simulink model "Test1"  (R2021b)
settings: Solver=FixedStepDiscrete  StartTime=0.0  StopTime=inf  RelTol=1e-3
undefined symbols (not defined in the file or in its folder): fdesignblkfcn, gcbh, High
libraries: dspswit3 x3, simulink x2, dspsnks4 x1, dspmtrx3 x1, dspvision x1, dspbuff3 x1, audiosources x1
settings Model: Creator=lenovo  LastModifiedBy=lenovo
settings SolverCC: AlgebraicLoopSolver=TrustRegion  AutoInsertRateTranBlk=on
settings DataIOCC: LimitDataPoints=on  SaveOutput=off  SignalLogging=off  SaveTime=off
settings OptimizationCC: LifeSpan=inf
settings DebuggingCC: AlgebraicLoopMsg=error  SingleTaskRateTransMsg=error  AllowSymbolicDim=off  SFUnexpectedBacktrackingDiag=warning  SFNoUnconditionalDefaultTransitionDiag=warning  SFExecutionAtInitializationDiag=none  SFMachineParentedDataDiag=warning  ArithmeticOperatorsInVariantConditions=warning
settings SFSimCC: SimUseLocalCustomCode=off  CustomCodeUndefinedFunction=UseInterfaceOnly
settings RTWCC: RTWUseLocalCustomCode=off
settings CodeAppCC: StateflowObjectComments=on
settings GRTTargetCC: TargetLangStandard=C89/C90 (ANSI)
settings ConfigComp: CovMetricSettings=dw  CovSaveCumulativeToWorkspaceVar=on  CovSaveSingleToWorkspaceVar=on  CovExternalEMLEnable=off  CovSFcnEnable=off

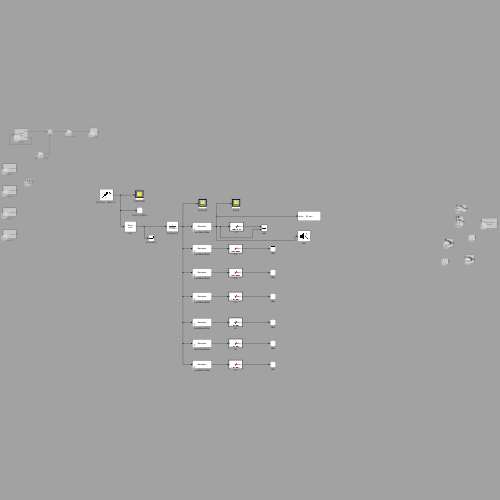
[thumbnail: Simulink's stored preview of the top-level diagram]
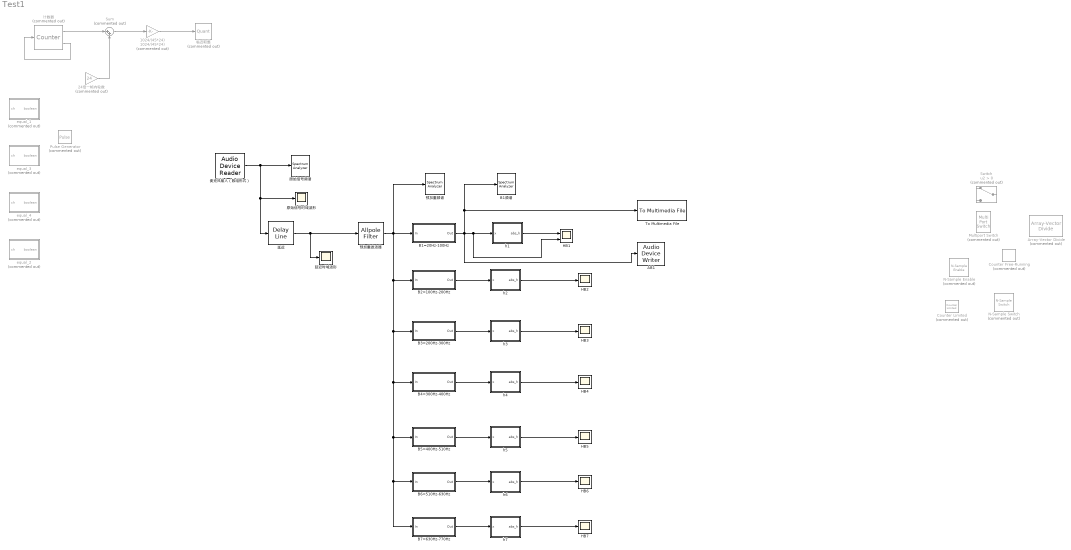
== system Test1 ==
  1024/(45*24) : Gain  Commented=on  Gain=1024/(45*24)
  24倍一帧内轮数 : Gain  Commented=on  Gain=24
  AB1 : dspsnks4/Audio Device Writer  Driver=DirectSound  Device=Default  InheritSampleRate=on  SampleRate=44100  BitDepth=16-bit integer  BufferSize=4096  NumBuffers=10  DefaultOutputChannelMapping=on  OutputChannelMapping=1:2  OutputNumUnderrunSamples=off  DriverIdx=1  DeviceWarnFlag=''
  Array-Vector Divide : dspmtrx3/Array-Vector Divide  Commented=on  Dimension=1  V_Source=Input port  V_VectFromMask=[0.5 0.25]  prodOutputSignedness=Auto  accumSignedness=Auto  roundingMode=Floor  overflowMode=off  firstCoeffSignedness=Auto  firstCoeffDataTypeStr=Inherit: Same word length as input  firstCoeffMin=[]  firstCoeffMax=[]  firstCoeffLastDataTypeStr=Inherit: Same word length as input  outputSignedness=Auto  outputMin=[]  outputMax=[]
      settings: SourceProductBaseCode=DS
  B1=20Hz-100Hz : Subsystem  DialogController=fdesignblkfcn  InitFcn=fdesignblkfcn(gcbh, {'InitFcn'});  mask(Bandpass Filter){}
      mask help: Design a bandpass filter
      settings: CopyFcn=fdesignblkfcn(gcbh, {'CopyFcn'});
      mask Help: helpview(mapfilelocation('dsp'), 'dspbandpassfilter');
      mask Display: disp('Bandpass');
  B1频谱 : SpectrumAnalyzer
  B2=100Hz-200Hz : Subsystem  DialogController=fdesignblkfcn  InitFcn=fdesignblkfcn(gcbh, {'InitFcn'});  mask(Bandpass Filter){}
      mask help: Design a bandpass filter
      settings: CopyFcn=fdesignblkfcn(gcbh, {'CopyFcn'});
      mask Help: helpview(mapfilelocation('dsp'), 'dspbandpassfilter');
      mask Display: disp('Bandpass');
  B3=200Hz-300Hz : Subsystem  DialogController=fdesignblkfcn  InitFcn=fdesignblkfcn(gcbh, {'InitFcn'});  mask(Bandpass Filter){}
      mask help: Design a bandpass filter
      settings: CopyFcn=fdesignblkfcn(gcbh, {'CopyFcn'});
      mask Help: helpview(mapfilelocation('dsp'), 'dspbandpassfilter');
      mask Display: disp('Bandpass');
  B4=300Hz-400Hz : Subsystem  DialogController=fdesignblkfcn  InitFcn=fdesignblkfcn(gcbh, {'InitFcn'});  mask(Bandpass Filter){}
      mask help: Design a bandpass filter
      settings: CopyFcn=fdesignblkfcn(gcbh, {'CopyFcn'});
      mask Help: helpview(mapfilelocation('dsp'), 'dspbandpassfilter');
      mask Display: disp('Bandpass');
  B5=400Hz-510Hz : Subsystem  DialogController=fdesignblkfcn  InitFcn=fdesignblkfcn(gcbh, {'InitFcn'});  mask(Bandpass Filter){}
      mask help: Design a bandpass filter
      settings: CopyFcn=fdesignblkfcn(gcbh, {'CopyFcn'});
      mask Help: helpview(mapfilelocation('dsp'), 'dspbandpassfilter');
      mask Display: disp('Bandpass');
  B6=510Hz-630Hz : Subsystem  DialogController=fdesignblkfcn  InitFcn=fdesignblkfcn(gcbh, {'InitFcn'});  mask(Bandpass Filter){}
      mask help: Design a bandpass filter
      settings: CopyFcn=fdesignblkfcn(gcbh, {'CopyFcn'});
      mask Help: helpview(mapfilelocation('dsp'), 'dspbandpassfilter');
      mask Display: disp('Bandpass');
  B7=630Hz-770Hz : Subsystem  DialogController=fdesignblkfcn  InitFcn=fdesignblkfcn(gcbh, {'InitFcn'});  mask(Bandpass Filter){}
      mask help: Design a bandpass filter
      settings: CopyFcn=fdesignblkfcn(gcbh, {'CopyFcn'});
      mask Help: helpview(mapfilelocation('dsp'), 'dspbandpassfilter');
      mask Display: disp('Bandpass');
  Counter Free-Running : simulink/Sources/Counter Free-Running  Commented=on  NumBits=16  tsamp=-1
  Counter Limited : simulink/Sources/Counter Limited  Commented=on  uplimit=7  tsamp=-1
  HB1 : Scope  NumInputPorts=2
  HB{2..7} (6 alike) : Scope
  Multiport Switch : MultiPortSwitch  Commented=on
  N-Sample Enable : dspswit3/N-Sample Enable  Commented=on  N=8  ActiveLevel=High (1)  reset=off  TriggerType=Rising edge  Ts=1  DataType=Logical
      settings: SourceProductBaseCode=DS
  N-Sample Switch : dspswit3/N-Sample Switch  Commented=on  N=8  reset=off  TriggerType=Rising edge  Ts=0.1
      settings: SourceProductBaseCode=DS
  Pulse Generator : DiscretePulseGenerator  Commented=on  PulseType=Time based  Period=10  PulseWidth=5
  Sum : Sum  Commented=on  Inputs=|++
  Switch : Switch  Commented=on  Criteria=u2 > Threshold
  To Multimedia File : dspvision/To Multimedia File  outputFilename=B1.wav  streamSelection=Audio only  videoCompressor=None (uncompressed)  audioCompressor=None (uncompressed)  imagePorts=Separate color signals  fileType=WAV  audioDatatype=16-bit integer  fourcc=RGB  videoQuality=75  mj2000CompFactor=10
  equal_1 : MATLAB Function  Commented=on  TreatAsAtomicUnit=on
  equal_2 : MATLAB Function  Commented=on  TreatAsAtomicUnit=on
  equal_3 : MATLAB Function  Commented=on  TreatAsAtomicUnit=on
  equal_4 : MATLAB Function  Commented=on  TreatAsAtomicUnit=on
  h1 : MATLAB Function  TreatAsAtomicUnit=on
  h2 : MATLAB Function  TreatAsAtomicUnit=on
  h3 : MATLAB Function  TreatAsAtomicUnit=on
  h4 : MATLAB Function  TreatAsAtomicUnit=on
  h5 : MATLAB Function  TreatAsAtomicUnit=on
  h6 : MATLAB Function  TreatAsAtomicUnit=on
  h7 : MATLAB Function  TreatAsAtomicUnit=on
  临近取整 : Quantizer  Commented=on  QuantizationInterval=1  LinearizeAsGain=off
  原始信号时域波形 : Scope
  原始信号频谱 : SpectrumAnalyzer
  延迟 : dspbuff3/Delay Line  siz=1024  ic=0  directfeed=off  enable_output=off  hold_output=off  OutputFrames=off
      settings: SourceProductBaseCode=DS
  延迟时域波形 : Scope
  计数器 : dspswit3/Counter  Commented=on  Direction=Up  CountEvent=Free running  CounterSize=User defined  MaxCount=25  InitialCount=1  Output=Count and Hit  HitValue=1  ResetInput=on  SamplesPerFrame=24*45  Ts=1/44100  CntDtype=double  HitDtype=Boolean
  预加重滤波器 : AllpoleFilter  Coefficients=[1 -0.95]
  预加重频谱 : SpectrumAnalyzer
  麦克风输入（数组形式） : audiosources/Audio Device Reader  Driver=DirectSound  Device=麦克风阵列 (适用于数字麦克风的英特尔? 智音技术)  SampleRate=44100  NumChannels=1  SamplesPerFrame=1024  BitDepth=16-bit integer  NumBuffers=10  DefaultInputChannelMapping=on  InputChannelMapping=1:2  OutputNumOverrunSamples=off  OutputDataType=double  DriverIdx=1  DeviceWarnFlag=''
      settings: SourceProductBaseCode=AU
  wires:
  麦克风输入（数组形式）/1 -> 原始信号时域波形/1, 延迟/1, 原始信号频谱/1
  延迟/1 -> 延迟时域波形/1, 预加重滤波器/1
  B1=20Hz-100Hz/1(Out) -> AB1/1, HB1/2, h1/1(x), B1频谱/1, To Multimedia File/1
  h1/1(abs_h) -> HB1/1
  B2=100Hz-200Hz/1(Out) -> h2/1(x)
  B3=200Hz-300Hz/1(Out) -> h3/1(x)
  B4=300Hz-400Hz/1(Out) -> h4/1(x)
  B5=400Hz-510Hz/1(Out) -> h5/1(x)
  B6=510Hz-630Hz/1(Out) -> h6/1(x)
  B7=630Hz-770Hz/1(Out) -> h7/1(x)
  h2/1(abs_h) -> HB2/1
  h3/1(abs_h) -> HB3/1
  h4/1(abs_h) -> HB4/1
  h5/1(abs_h) -> HB5/1
  h6/1(abs_h) -> HB6/1
  h7/1(abs_h) -> HB7/1
  计数器/2 -> 计数器/1
  计数器/1 -> Sum/1
  24倍一帧内轮数/1 -> Sum/2
  Sum/1 -> 1024/(45*24)/1
  1024/(45*24)/1 -> 临近取整/1
  预加重滤波器/1 -> B7=630Hz-770Hz/1(In), B6=510Hz-630Hz/1(In), B5=400Hz-510Hz/1(In), B4=300Hz-400Hz/1(In), B3=200Hz-300Hz/1(In), B2=100Hz-200Hz/1(In), 预加重频谱/1, B1=20Hz-100Hz/1(In)

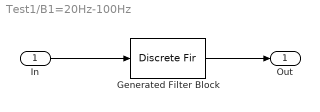
== system Test1/B1=20Hz-100Hz ==
  In : Inport
  Generated Filter Block : DiscreteFir  Tag=BlockMethodSubSystem  Coefficients=[0.00457402244520528894 0.00508602619083937946 0.00659269331412791308 0.00903956144930821194 0.0123353711920271541 0.016355548458740897 0.0209470008592822429 0.0259340418292448825 0.0311252113312927223 0.0363207260934495305 0.0413202670506143815 0.0459307979165471392 0.0499741072000983652 0.0532937765702380661 0.0557613008604806379 0.0572811183038447469 0.0577943524869048084 0.0572811183038447469 0.0557613008604806379 0.0532937765702380661 0.0499741072000983652 0.0459307979165471392 0.0413202670506143815 0.0363207260934495305 0.0311252113312927223 0.0259340418292448825 0.0209470008592822429 0.016355548458740897 0.0123353711920271541 0.00903956144930821194 0.00659269331412791308 0.00508602619083937946 0.00457402244520528894]  InputProcessing=Columns as channels (frame based)
  Out : Outport  VectorParamsAs1DForOutWhenUnconnected=off
  wires:
  In/1 -> Generated Filter Block/1
  Generated Filter Block/1 -> Out/1

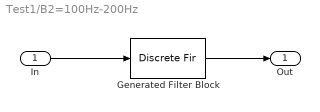
== system Test1/B2=100Hz-200Hz ==
  In : Inport
  Generated Filter Block : DiscreteFir  Tag=BlockMethodSubSystem  Coefficients=[0.00441727693112917499 0.0049428047170021602 0.00644474326614278507 0.00888485385185234372 0.0121851336333958435 0.0162306434727095723 0.0208739501835365493 0.0259410032521986307 0.0312382012424146337 0.0365603488452490091 0.0416991643701427883 0.0464519713170962745 0.0506301977683168147 0.0540673141973552276 0.0566258636594231327 0.0582032771897738541 0.0587362198811968786 0.0582032771897738541 0.0566258636594231327 0.0540673141973552276 0.0506301977683168147 0.0464519713170962745 0.0416991643701427883 0.0365603488452490091 0.0312382012424146337 0.0259410032521986307 0.0208739501835365493 0.0162306434727095723 0.0121851336333958435 0.00888485385185234372 0.00644474326614278507 0.0049428047170021602 0.00441727693112917499]  InputProcessing=Columns as channels (frame based)
  Out : Outport  VectorParamsAs1DForOutWhenUnconnected=off
  wires:
  In/1 -> Generated Filter Block/1
  Generated Filter Block/1 -> Out/1

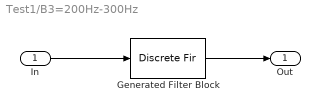
== system Test1/B3=200Hz-300Hz ==
  In : Inport
  Generated Filter Block : DiscreteFir  Tag=BlockMethodSubSystem  Coefficients=[0.0040814662241728597 0.00463418043527237707 0.00612377247553548727 0.00854634110797388227 0.0118523009197635167 0.0159476618531074477 0.02069756837227818 0.0259319465742560012 0.0314529964840676579 0.0370441687734499453 0.0424801854503906937 0.0475376069779057803 0.0520054168949762724 0.0556950910760549422 0.0584496425706742123 0.0601511833336923971 0.060726618501989918 0.0601511833336923971 0.0584496425706742123 0.0556950910760549422 0.0520054168949762724 0.0475376069779057803 0.0424801854503906937 0.0370441687734499453 0.0314529964840676579 0.0259319465742560012 0.02069756837227818 0.0159476618531074477 0.0118523009197635167 0.00854634110797388227 0.00612377247553548727 0.00463418043527237707 0.0040814662241728597]  InputProcessing=Columns as channels (frame based)
  Out : Outport  VectorParamsAs1DForOutWhenUnconnected=off
  wires:
  In/1 -> Generated Filter Block/1
  Generated Filter Block/1 -> Out/1

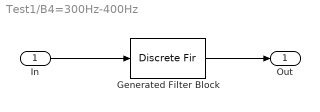
== system Test1/B4=300Hz-400Hz ==
  In : Inport
  Generated Filter Block : DiscreteFir  Tag=BlockMethodSubSystem  Coefficients=[0.00355254435048634127 0.00414283836891639941 0.00560631324623054542 0.0079917846773801017 0.0112942797519545203 0.0154535136154739811 0.0203556333711287542 0.0258381626345098731 0.031697887414365189 0.0377012460605533825 0.0435966336799673629 0.0491279139259522268 0.0540483555780169253 0.0581341824796804546 0.0611969450154634734 0.0630939882821951181 0.0637364024848837418 0.0630939882821951181 0.0611969450154634734 0.0581341824796804546 0.0540483555780169253 0.0491279139259522268 0.0435966336799673629 0.0377012460605533825 0.031697887414365189 0.0258381626345098731 0.0203556333711287542 0.0154535136154739811 0.0112942797519545203 0.0079917846773801017 0.00560631324623054542 0.00414283836891639941 0.00355254435048634127]  InputProcessing=Columns as channels (frame based)
  Out : Outport  VectorParamsAs1DForOutWhenUnconnected=off
  wires:
  In/1 -> Generated Filter Block/1
  Generated Filter Block/1 -> Out/1

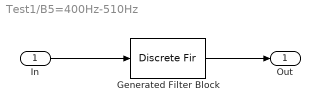
== system Test1/B5=400Hz-510Hz ==
  In : Inport
  Generated Filter Block : DiscreteFir  Tag=BlockMethodSubSystem  Coefficients=[0.00275971456380242003 0.00339533901013880585 0.00480565315502284353 0.0071156523803956517 0.0103869854100731001 0.0146114696892858317 0.0197093465287720912 0.0255324304760224559 0.0318719740834857643 0.0384707474251257744 0.0450385433246698191 0.0512700839953592266 0.0568641387387727182 0.0615425768889026961 0.0650680812105939727 0.0672593344715345098 0.0680026600138681353 0.0672593344715345098 0.0650680812105939727 0.0615425768889026961 0.0568641387387727182 0.0512700839953592266 0.0450385433246698191 0.0384707474251257744 0.0318719740834857643 0.0255324304760224559 0.0197093465287720912 0.0146114696892858317 0.0103869854100731001 0.0071156523803956517 0.00480565315502284353 0.00339533901013880585 0.00275971456380242003]  InputProcessing=Columns as channels (frame based)
  Out : Outport  VectorParamsAs1DForOutWhenUnconnected=off
  wires:
  In/1 -> Generated Filter Block/1
  Generated Filter Block/1 -> Out/1

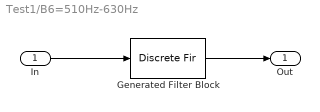
== system Test1/B6=510Hz-630Hz ==
  In : Inport
  Generated Filter Block : DiscreteFir  Tag=BlockMethodSubSystem  Coefficients=[0.00158038072817055244 0.0022616527536898582 0.00356511150029509933 0.0057235260776234663 0.00889731727110634057 0.0131592040400760682 0.0184856459001761127 0.0247557734984594907 0.0317579235027212262 0.0392033081399341676 0.0467457994294747728 0.0540063357554068715 0.0606001003233641242 0.0661644048821167785 0.0703851545710504067 0.0730198753867326716 0.0739155464885860036 0.0730198753867326716 0.0703851545710504067 0.0661644048821167785 0.0606001003233641242 0.0540063357554068715 0.0467457994294747728 0.0392033081399341676 0.0317579235027212262 0.0247557734984594907 0.0184856459001761127 0.0131592040400760682 0.00889731727110634057 0.0057235260776234663 0.00356511150029509933 0.0022616527536898582 0.00158038072817055244]  InputProcessing=Columns as channels (frame based)
  Out : Outport  VectorParamsAs1DForOutWhenUnconnected=off
  wires:
  In/1 -> Generated Filter Block/1
  Generated Filter Block/1 -> Out/1

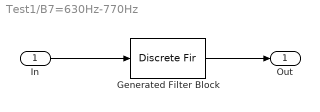
== system Test1/B7=630Hz-770Hz ==
  In : Inport
  Generated Filter Block : DiscreteFir  Tag=BlockMethodSubSystem  Coefficients=[-0.000162676716799283665 0.000541779660954365395 0.00163064713593765852 0.00348488591192890832 0.00641064109455515355 0.0106078367437588764 0.0161481471425824301 0.0229643237517662413 0.0308518627852202576 0.0394829173921623297 0.0484312847250816178 0.0572063258000772776 0.0652928902875049288 0.0721937881687217536 0.0774711221555558216 0.0807828890253932119 0.0819116664682331963 0.0807828890253932119 0.0774711221555558216 0.0721937881687217536 0.0652928902875049288 0.0572063258000772776 0.0484312847250816178 0.0394829173921623297 0.0308518627852202576 0.0229643237517662413 0.0161481471425824301 0.0106078367437588764 0.00641064109455515355 0.00348488591192890832 0.00163064713593765852 0.000541779660954365395 -0.000162676716799283665]  InputProcessing=Columns as channels (frame based)
  Out : Outport  VectorParamsAs1DForOutWhenUnconnected=off
  wires:
  In/1 -> Generated Filter Block/1
  Generated Filter Block/1 -> Out/1

== matlab function Test1/h1 ==
  data: x input; abs_h output
function abs_h = reorganise(x)
    N=1024;
    Z=complex(1,1)*zeros(N,1);
    X=fft(x);
    Z(1)=X(1);
    Z(2:N/2)=2*X(2:N/2);
    Z(N/2+1:N)=0;
    z=imag(ifft(Z));
    abs_h=sqrt(z.*z+x.*x);

== matlab function Test1/h3 ==
  data: x input; abs_h output
function abs_h = reorganise(x)
    N=1024;
    Z=complex(1,1)*zeros(N,1);
    X=fft(x);
    Z(1)=X(1);
    Z(2:N/2)=2*X(2:N/2);
    Z(N/2+1:N)=0;
    z=imag(ifft(Z));
    abs_h=sqrt(z.*z+x.*x);

== matlab function Test1/h4 ==
  data: x input; abs_h output
function abs_h = reorganise(x)
    N=1024;
    Z=complex(1,1)*zeros(N,1);
    X=fft(x);
    Z(1)=X(1);
    Z(2:N/2)=2*X(2:N/2);
    Z(N/2+1:N)=0;
    z=imag(ifft(Z));
    abs_h=sqrt(z.*z+x.*x);

== matlab function Test1/h5 ==
  data: x input; abs_h output
function abs_h = reorganise(x)
    N=1024;
    Z=complex(1,1)*zeros(N,1);
    X=fft(x);
    Z(1)=X(1);
    Z(2:N/2)=2*X(2:N/2);
    Z(N/2+1:N)=0;
    z=imag(ifft(Z));
    abs_h=sqrt(z.*z+x.*x);

== matlab function Test1/h6 ==
  data: x input; abs_h output
function abs_h = reorganise(x)
    N=1024;
    Z=complex(1,1)*zeros(N,1);
    X=fft(x);
    Z(1)=X(1);
    Z(2:N/2)=2*X(2:N/2);
    Z(N/2+1:N)=0;
    z=imag(ifft(Z));
    abs_h=sqrt(z.*z+x.*x);

== matlab function Test1/h7 ==
  data: x input; abs_h output
function abs_h = reorganise(x)
    N=1024;
    Z=complex(1,1)*zeros(N,1);
    X=fft(x);
    Z(1)=X(1);
    Z(2:N/2)=2*X(2:N/2);
    Z(N/2+1:N)=0;
    z=imag(ifft(Z));
    abs_h=sqrt(z.*z+x.*x);

== matlab function Test1/equal_1 ==
  data: ch input; boolean output
function boolean = equal_1(ch)
%#codegen
if ch==1
    boolean=1;
else
    boolean=0;
end

== matlab function Test1/equal_2 ==
  data: ch input; boolean output
function boolean = equal_2(ch)
%#codegen
if ch==2
    boolean=1;
else
    boolean=0;
end

== matlab function Test1/h2 ==
  data: x input; abs_h output
function abs_h = reorganise(x)
    N=1024;
    Z=complex(1,1)*zeros(N,1);
    X=fft(x);
    Z(1)=X(1);
    Z(2:N/2)=2*X(2:N/2);
    Z(N/2+1:N)=0;
    z=imag(ifft(Z));
    abs_h=sqrt(z.*z+x.*x);

== matlab function Test1/equal_3 ==
  data: ch input; boolean output
function boolean = equal_3(ch)
%#codegen
if ch==3
    boolean=1;
else
    boolean=0;
end

== matlab function Test1/equal_4 ==
  data: ch input; boolean output
function boolean = equal_4(ch)
%#codegen
if ch==4
    boolean=1;
else
    boolean=0;
end
